simulink model "ArduinoSubsystem"  (R2019a)
settings: Solver=VariableStepAuto  StartTime=0.0  StopTime=inf  RelTol=1e-3
InitFcn:
  | stringToSend = "Hello";
  | prevString = "";
model workspace (MAT data in the model file):
  Period = Simulink.Signal
  Period.DataType = 'auto'
  Period.Dimensions = -1
  Period.DimensionsMode = 'auto'
  Period.Complexity = 'auto'
  Period.SampleTime = 0.5
  Period.SamplingMode = 'auto'
  Period.InitialValue = '0.5'
undefined symbols (not defined in the file or in its folder): LF
libraries: instrumentlib x3, etargetslib x1
settings Model: EnablePacing=on  OrderedModelArguments=off  Creator=Julien  LastModifiedBy=Julien
settings DebuggingCC: SFMachineParentedDataDiag=error

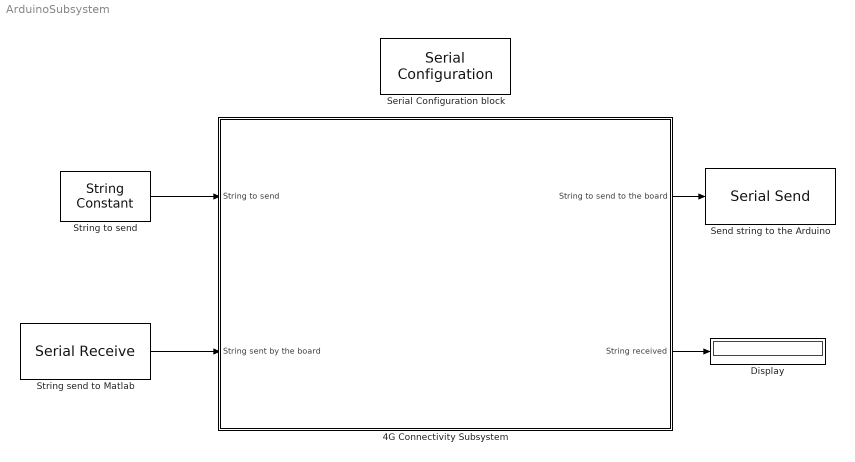
== system ArduinoSubsystem ==
  4G Connectivity Subsystem : Subsystem
  Display : Display
  Send string to the Arduino : instrumentlib/Serial Send  Priority=1  ObjConstructor=serial('<Select a port...>');  ComPortMenu=<Please select a port...>  ComPort=<Please select a port...>  Terminator=LF ('\n')  EnableBlockingMode=off
  Serial Configuration block : instrumentlib/Serial Configuration  Priority=-200000  ObjConstructor=serial('<Select a port...>');  ComPortMenu=<Please select a port...>  ComPort=<Please select a port...>  BaudRate=57600  DataBits=8  Parity=none  StopBits=1  ByteOrder=LittleEndian  FlowControl=none  Timeout=10
  String send to Matlab : instrumentlib/Serial Receive  Priority=1  ObjConstructor=serial('<Select a port...>');  ComPortMenu=<Please select a port...>  ComPort=<Please select a port...>  DataType=uint8  Terminator=LF ('\n')  DataSize=[1 10]  EnableBlockingMode=on  ActionDataUnavailable=Output last received value  CustomValue=0  SampleTime=0.3
  String to send : StringConstant  String=stringToSend
  wires:
  4G Connectivity Subsystem/1(String to send to the board) -> Send string to the Arduino/1
  String send to Matlab/1 -> 4G Connectivity Subsystem/2(String sent by the board)
  4G Connectivity Subsystem/2(String received) -> Display/1
  String to send/1 -> 4G Connectivity Subsystem/1(String to send)

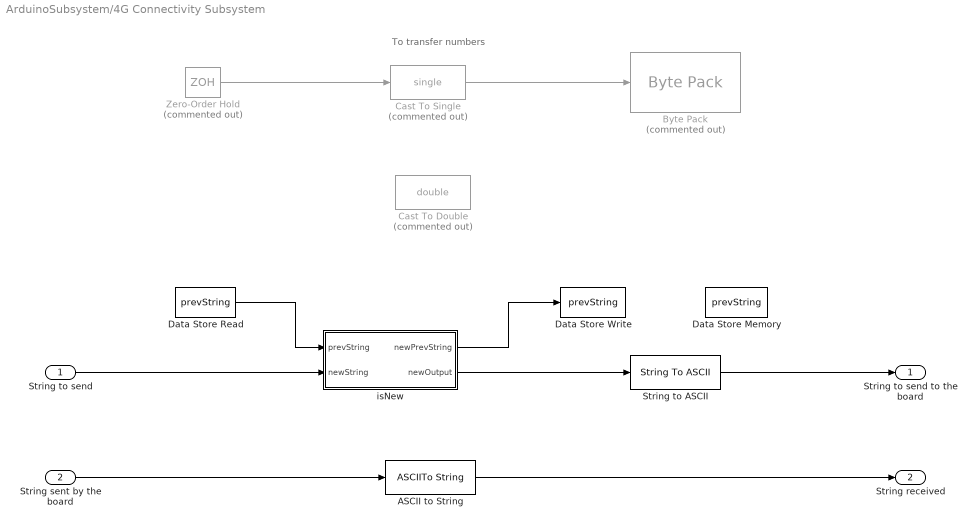
== system ArduinoSubsystem/4G Connectivity Subsystem ==
  note: To transfer numbers
  String to send : Inport
  String sent by the board : Inport  Port=2
  ASCII to String : ASCIIToString
  Byte Pack : etargetslib/Byte Pack  Commented=on  datatypes={'single'}  byteAlign=4
  Cast To Double : DataTypeConversion  Commented=on  OutDataTypeStr=double
  Cast To Single : DataTypeConversion  Commented=on  OutDataTypeStr=single
  Data Store Memory : DataStoreMemory  DataStoreName=prevString  ReadBeforeWriteMsg=warning  WriteAfterWriteMsg=warning  WriteAfterReadMsg=warning  ShowAdditionalParam=off  OutDataTypeStr=string
  Data Store Read : DataStoreRead  DataStoreName=prevString  DataStoreElements=prevString
  Data Store Write : DataStoreWrite  DataStoreName=prevString  DataStoreElements=prevString
  String to ASCII : StringToASCII  OutputVectorSize=10
  Zero-Order Hold : ZeroOrderHold  Commented=on  SampleTime=0.3
  isNew : MATLAB Function  TreatAsAtomicUnit=on
  String to send to the board : Outport
  String received : Outport  Port=2
  wires:
  Cast To Single/1 -> Byte Pack/1
  Zero-Order Hold/1 -> Cast To Single/1
  String sent by the board/1 -> ASCII to String/1
  ASCII to String/1 -> String received/1
  Data Store Read/1 -> isNew/1(prevString)
  isNew/1(newPrevString) -> Data Store Write/1
  String to send/1 -> isNew/2(newString)
  isNew/2(newOutput) -> String to ASCII/1
  String to ASCII/1 -> String to send to the board/1

== matlab function ArduinoSubsystem/4G Connectivity Subsystem/isNew ==
  data: prevString input; newPrevString output; newString input; newOutput output
function [newPrevString,newOutput] = isNew(prevString, newString)
    newOutput = "";
    newPrevString = prevString;
    if(newString ~= prevString)
        newOutput = newString;
        newPrevString = newString;
    end
end
